simulink model "mpc555_v12_sade_ve_duzenli"  (Simulink 7.0)
settings: Solver=FixedStepDiscrete  StartTime=0.0  StopTime=inf  FixedStep=dt_sys  RelTol=1e-3
PreLoadFcn:
  | RTWConfigurationCB('preloadfcn', bdroot);
InitFcn:
  | % START RTW CONFIGURATION CODE %
  | RTWConfigurationCB('rtw_target_initfcn',gcs);
  | % END RTW CONFIGURATION CODE %
values from neighbouring files (symbols this model uses):
  dt = 1/50    (= 0.02)    [init_par.m]
  dt_serial_RX1 = dt/120    (= 0.000166666666667)    [init_par.m]
  dt_serial_TX2 = dt/120    (= 0.000166666666667)    [init_par.m]
undefined symbols (not defined in the file or in its folder): DiscIntNeverNeededParam
libraries: aerolibconvert2 x9, mpc555drivers x5, simulink x1
(part 1 of 2)
settings Model: Creator=PC  LastModifiedBy=eg
settings OptimizationCC: OptimizeModelRefInitCode=on  LifeSpan=1
settings DebuggingCC: AlgebraicLoopMsg=none
settings HardwareCC: ProdIntDivRoundTo=Zero  ProdEndianess=BigEndian  ProdHWDeviceType=Motorola PowerPC
settings RTWCC: SystemTargetFile=mpc555rt.tlc  TemplateMakefile=mpc555rt.tmf  Description=Target for Freescale MPC5xx (real-time)  ProcessScript=mpc555rt_make_rtw_hook
settings CodeAppCC: IgnoreCustomStorageClasses=off
settings STFCustomTargetCC: TargetLibSuffix=.a  TargetPreCompLibLocation=C:\MATLAB\R2007b\toolbox\rtw\targets\mpc555dk\drivers\lib\CODE_WARRIOR  GenFloatMathFcnCalls=ANSI_C  IncludeMdlTerminateFcn=off  CombineOutputUpdateFcns=on  ERTCustomFileBanners=on  SupportNonFinite=off  SupportContinuousTime=off  SupportNonInlinedSFcns=off  SystemTargetFile=mpc555rt.tlc
settings ERTTargetCC: TargetPreCompLibLocation=C:\MATLAB\R2007b\toolbox\rtw\targets\mpc555dk\drivers\lib\CODE_WARRIOR  GenFloatMathFcnCalls=ANSI_C  CompOptLevelCompliant=off  IncludeMdlTerminateFcn=off  SupportNonFinite=off  ModelStepFunctionPrototypeControlCompliant=off  ExtModeMexFile=MPC5xxExternalModeOpen  ExtModeIntrfLevel=Level2 - Open  InlinedParameterPlacement=NonHierarchical  ERTCustomFileTemplate=example_file_process.tlc
settings CustomProperty: DataType=RTWOptions_EnumType__toolbox_rtw_targets_mpc555dk_mpc555dk_mpc555rt_MPC555_OPTIMIZATION_SWITCH  Value=speed
settings EnumStrPairs: String=speed

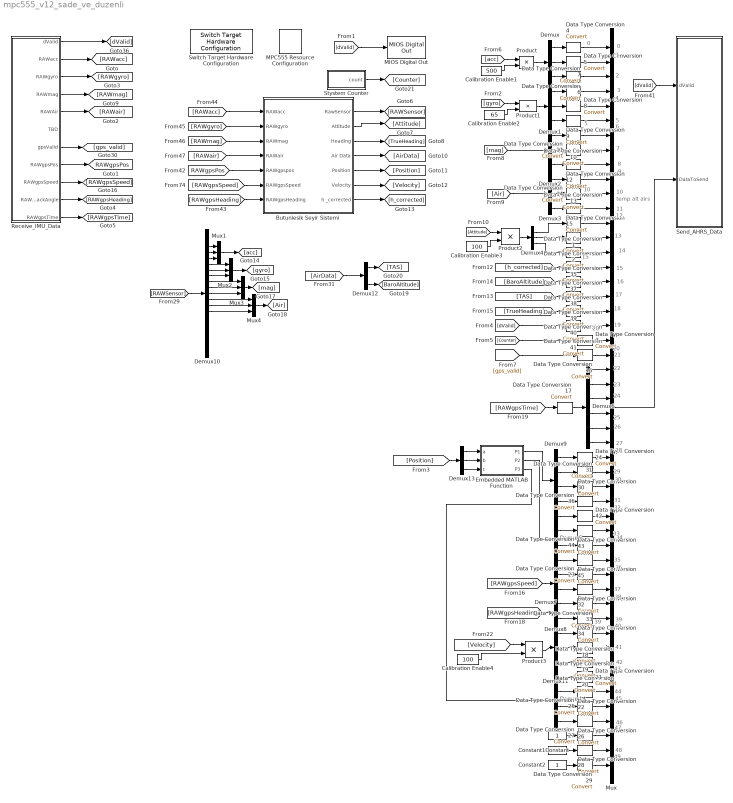
== system mpc555_v12_sade_ve_duzenli ==
  note: 0
  note: 5
  note: 10
  note: 15
  note: 20
  note: 39
  note: 27
  note: 0
  note: 1
  note: 2
  note: 4
  note: 5
  note: 6
  note: 7
  note: 8
  note: 9
  note: 10
  note: 11
  note: 12
  note: 13
  note: 14
  note: 15
  note: 16
  note: 3
  note: 17
  note: 18
  note: 19
  note: 20
  note: 21
  note: 22
  note: 23
  note: 24
  note: 25
  note: 26
  note: 28
  note: 29
  note: 30
  note: 31
  note: 32
  note: 33
  note: 34
  note: 35
  note: 36
  note: 37
  note: 38
  note: 39
  note: 40
  note: 41
  note: 42
  note: 43
  note: 44
  note: 45
  note: 46
  note: 47
  note: 48
  note: 49
  note: temp
      | alt
      | airs
  Butunlesik Seyir Sistemi : Subsystem
  Calibration Enable1 : Constant  Value=500  OutDataType=fixdt(1, 16)  OutScaling=2^0
  Calibration Enable2 : Constant  Value=65  OutDataType=fixdt(1, 16)  OutScaling=2^0
  Calibration Enable3 : Constant  Value=100  OutDataType=fixdt(1, 16)  OutScaling=2^0
  Calibration Enable4 : Constant  Value=100  OutDataType=fixdt(1, 16)  OutScaling=2^0
  Constant : Constant  OutDataType=sfix(16)  OutScaling=2^0
  Constant1 : Constant  OutDataType=sfix(16)  OutScaling=2^0
  Constant2 : Constant  OutDataType=sfix(16)  OutScaling=2^0
  Data Type Conversion{1..45} (45 alike) : DataTypeConversion  OutDataTypeMode=int16  OutDataType=sfix(16)  OutScaling=2^0
  Demux{,1..4,11,13} (7 alike) : Demux  Outputs=3
  Demux10 : Demux  Outputs=17
  Demux{5,9,12,14} (4 alike) : Demux
  Demux6 : Demux  Outputs=6
  Demux7 : Demux  Outputs=2
  Demux8 : Demux  Outputs=2
  Embedded MATLAB Function : Stateflow chart
  MIOS Digital Out : mpc555drivers/Modular Input//Output System (MIOS1)/MIOS Digital Out  SystemSampleTime=-1  bits=[3]  init=0  t=-1  enablePassThru=off
  MPC555 Resource Configuration : mpc555drivers/MPC555 Resource Configuration  Tag=RTW CONFIGURATION BLOCK  Priority=-100000  SystemSampleTime=-1  oldParentName=mpc555_v12_sade_ve_duzenli  oldBlockName=|
      | mpc555_v12_sade_ve_duzenli/MPC555
      | Resource
      | Configuration
  Mux : Mux  Inputs=50
  Mux{1..4} (4 alike) : Mux  Inputs=3
  Product{,1..3} (4 alike) : Product  OutDataType=sfix(16)  OutScaling=2^0  RndMeth=Zero
      mask Display: text(0.5, 0.5, ['SCI' num2str(module) '\nTransmit'],'horizontalAlignment','center'); port_label('input',1,'Data'); port_label('input', 2, 'Req');
  Receive_IMU_Data : Subsystem
  Send_AHRS_Data : Subsystem
  Stystem Counter : Stateflow chart
  Switch Target Hardware Configuration : mpc555drivers/Utilities/Switch Target Hardware Configuration  SystemSampleTime=-1
  tag scope: RAWgpsPos=global
  wires:
  Mux/1 -> Send_AHRS_Data/2(DataToSend)
  Data Type Conversion4/1 -> Mux/1
  Data Type Conversion5/1 -> Mux/2
  Data Type Conversion6/1 -> Mux/3
  Data Type Conversion7/1 -> Mux/4
  Data Type Conversion8/1 -> Mux/5
  Data Type Conversion9/1 -> Mux/6
  Data Type Conversion10/1 -> Mux/7
  Data Type Conversion11/1 -> Mux/8
  Data Type Conversion12/1 -> Mux/9
  Data Type Conversion13/1 -> Mux/10
  Data Type Conversion14/1 -> Mux/11
  Data Type Conversion15/1 -> Mux/12
  Data Type Conversion3/1 -> Mux/21
  Data Type Conversion16/1 -> Mux/22
  Demux6/2 -> Mux/24
  Data Type Conversion37/1 -> Mux/16
  Data Type Conversion38/1 -> Mux/17
  Data Type Conversion39/1 -> Mux/18
  Data Type Conversion40/1 -> Mux/19
  Data Type Conversion41/1 -> Mux/20
  Data Type Conversion23/1 -> Mux/37
  Data Type Conversion32/1 -> Mux/38
  Data Type Conversion33/1 -> Mux/39
  Data Type Conversion34/1 -> Mux/40
  [dValid] -> Send_AHRS_Data/1(dValid)
  Receive_IMU_Data/1(dValid) -> [dValid]
  Receive_IMU_Data/7(gpsValid) -> [gps_valid]
  Receive_IMU_Data/2(RAWacc) -> [RAWacc]
  Receive_IMU_Data/3(RAWgyro) -> [RAWgyro]
  Receive_IMU_Data/4(RAWmag) -> [RAWmag]
  Receive_IMU_Data/5(RAWAir) -> [RAWair]
  Receive_IMU_Data/8(RAWgpsPos) -> [RAWgpsPos]
  Receive_IMU_Data/9(RAWgpsSpeed) -> [RAWgpsSpeed]
  Receive_IMU_Data/10(RAWgpsTrackAngle) -> [RAWgpsHeading]
  Receive_IMU_Data/11(RAWgpsTime) -> [RAWgpsTime]
  Demux/1 -> Data Type Conversion4/1
  Demux/2 -> Data Type Conversion5/1
  [Air] -> Demux3/1
  Demux1/1 -> Data Type Conversion7/1
  Demux1/2 -> Data Type Conversion8/1
  Demux1/3 -> Data Type Conversion9/1
  Demux3/1 -> Data Type Conversion13/1
  Demux3/2 -> Data Type Conversion14/1
  Demux3/3 -> Data Type Conversion15/1
  Data Type Conversion1/1 -> Mux/13
  Data Type Conversion2/1 -> Mux/14
  Data Type Conversion35/1 -> Mux/15
  Demux4/1 -> Data Type Conversion1/1
  Demux4/2 -> Data Type Conversion2/1
  Demux4/3 -> Data Type Conversion35/1
  [RAWgpsHeading] -> Demux8/1
  Demux8/2 -> Data Type Conversion34/1
  Demux8/1 -> Data Type Conversion33/1
  Demux7/2 -> Data Type Conversion32/1
  Demux7/1 -> Data Type Conversion23/1
  [RAWgpsSpeed] -> Demux7/1
  Demux6/6 -> Mux/28
  Demux6/5 -> Mux/27
  Demux6/4 -> Mux/26
  Demux6/3 -> Mux/25
  [RAWgpsTime] -> Data Type Conversion17/1
  [h_corrected] -> Data Type Conversion37/1
  [BaroAltitude] -> Data Type Conversion38/1
  [TAS] -> Data Type Conversion39/1
  [dValid] -> Data Type Conversion41/1
  Product2/1 -> Demux4/1
  [Attitude] -> Product2/1
  Calibration Enable3/1 -> Product2/2
  Demux9/1 -> Data Type Conversion24/1
  Demux9/2 -> Data Type Conversion30/1
  Demux9/3 -> Data Type Conversion31/1
  Demux9/4 -> Data Type Conversion36/1
  Demux5/2 -> Data Type Conversion43/1
  Demux5/3 -> Data Type Conversion44/1
  Demux5/4 -> Data Type Conversion45/1
  Data Type Conversion17/1 -> Demux6/1
  Demux6/1 -> Mux/23
  Data Type Conversion18/1 -> Mux/41
  Data Type Conversion19/1 -> Mux/42
  Data Type Conversion20/1 -> Mux/43
  Data Type Conversion21/1 -> Mux/44
  Data Type Conversion22/1 -> Mux/45
  Data Type Conversion25/1 -> Mux/46
  Data Type Conversion26/1 -> Mux/47
  [RAWacc] -> Butunlesik Seyir Sistemi/1(RAWacc)
  [RAWgyro] -> Butunlesik Seyir Sistemi/2(RAWgyro)
  [RAWmag] -> Butunlesik Seyir Sistemi/3(RAWmag)
  [RAWair] -> Butunlesik Seyir Sistemi/4(RAWair)
  [RAWgpsPos] -> Butunlesik Seyir Sistemi/5(RAWgpspos)
  [RAWgpsSpeed] -> Butunlesik Seyir Sistemi/6(RAWgpsSpeed)
  [RAWgpsHeading] -> Butunlesik Seyir Sistemi/7(RAWgpsHeading)
  Butunlesik Seyir Sistemi/1(RawSensor) -> [RAWSensor]
  Butunlesik Seyir Sistemi/2(Attitude) -> [Attitude]
  Butunlesik Seyir Sistemi/3(Heading) -> [TrueHeading]
  Butunlesik Seyir Sistemi/4(Air Data) -> [AirData]
  Butunlesik Seyir Sistemi/5(Position) -> [Position]
  Butunlesik Seyir Sistemi/6(Velocity) -> [Velocity]
  Butunlesik Seyir Sistemi/7(h _corrected) -> [h_corrected]
  [RAWSensor] -> Demux10/1
  Demux10/1 -> Mux1/1
  Demux10/2 -> Mux1/2
  Demux10/3 -> Mux1/3
  Mux1/1 -> [acc]
  Mux2/1 -> [gyro]
  Demux10/4 -> Mux2/1
  Demux10/5 -> Mux2/2
  Demux10/6 -> Mux2/3
  Mux3/1 -> [mag]
  Demux10/7 -> Mux3/1
  Demux10/8 -> Mux3/2
  Demux10/9 -> Mux3/3
  Mux4/1 -> [Air]
  Demux10/10 -> Mux4/1
  Demux10/11 -> Mux4/2
  Demux10/12 -> Mux4/3
  [AirData] -> Demux12/1
  Demux12/4 -> [BaroAltitude]
  Demux12/1 -> [TAS]
  Data Type Conversion27/1 -> Mux/48
  Data Type Conversion28/1 -> Mux/49
  Data Type Conversion29/1 -> Mux/50
  [dValid] -> MIOS Digital Out/1
  Demux/3 -> Data Type Conversion6/1
  Product/1 -> Demux/1
  [acc] -> Product/1
  Calibration Enable1/1 -> Product/2
  [gyro] -> Product1/1
  Calibration Enable2/1 -> Product1/2
  Product1/1 -> Demux1/1
  Demux2/1 -> Data Type Conversion10/1
  Demux2/2 -> Data Type Conversion11/1
  Demux2/3 -> Data Type Conversion12/1
  Embedded MATLAB Function/1(P1) -> Demux9/1
  Embedded MATLAB Function/2(P2) -> Demux5/1
  Demux5/1 -> Data Type Conversion42/1
  [Velocity] -> Product3/1
  Calibration Enable4/1 -> Product3/2
  Product3/1 -> Demux11/1
  Data Type Conversion24/1 -> Mux/29
  Data Type Conversion30/1 -> Mux/30
  Data Type Conversion31/1 -> Mux/31
  Data Type Conversion36/1 -> Mux/32
  Data Type Conversion42/1 -> Mux/33
  Data Type Conversion43/1 -> Mux/34
  Data Type Conversion44/1 -> Mux/35
  Data Type Conversion45/1 -> Mux/36
  [Position] -> Demux13/1
  Demux11/1 -> Data Type Conversion18/1
  Demux11/2 -> Data Type Conversion19/1
  Demux11/3 -> Data Type Conversion20/1
  Stystem Counter/1(count) -> [Counter]
  [Counter] -> Data Type Conversion3/1
  [gps_valid] -> Data Type Conversion16/1
  Embedded MATLAB Function/3(P3) -> Demux14/1
  Demux14/1 -> Data Type Conversion21/1
  Demux14/2 -> Data Type Conversion22/1
  Demux14/3 -> Data Type Conversion25/1
  Demux14/4 -> Data Type Conversion26/1
  Constant/1 -> Data Type Conversion27/1
  Constant1/1 -> Data Type Conversion28/1
  Constant2/1 -> Data Type Conversion29/1
  Demux13/2 -> Embedded MATLAB Function/2(b)
  [mag] -> Demux2/1
  Demux13/1 -> Embedded MATLAB Function/1(a)
  Demux13/3 -> Embedded MATLAB Function/3(c)
  [TrueHeading] -> Data Type Conversion40/1

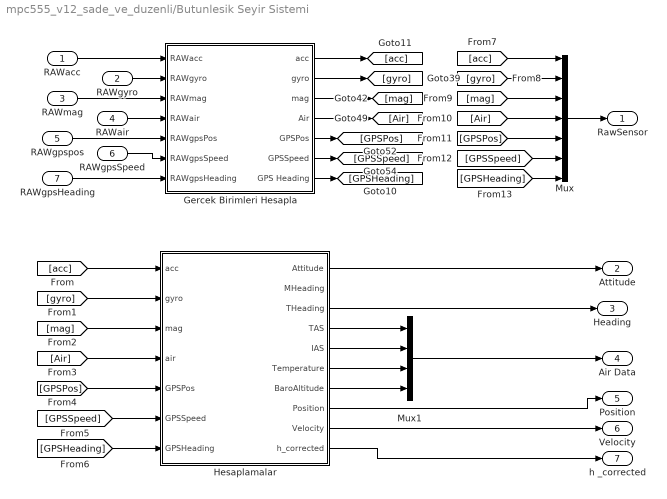
== system mpc555_v12_sade_ve_duzenli/Butunlesik Seyir Sistemi ==
  RAWacc : Inport  OutDataType=fixdt(1, 16)  OutScaling=2^0
  RAWgyro : Inport  Port=2  OutDataType=fixdt(1, 16)  OutScaling=2^0
  RAWmag : Inport  Port=3  OutDataType=fixdt(1, 16)  OutScaling=2^0
  RAWair : Inport  Port=4  OutDataType=fixdt(1, 16)  OutScaling=2^0
  RAWgpspos : Inport  Port=5  OutDataType=fixdt(1, 16)  OutScaling=2^0
  RAWgpsSpeed : Inport  Port=6  OutDataType=fixdt(1, 16)  OutScaling=2^0
  RAWgpsHeading : Inport  Port=7  OutDataType=fixdt(1, 16)  OutScaling=2^0
  Gercek Birimleri Hesapla : Subsystem
  Hesaplamalar : Subsystem
  Mux : Mux  Inputs=7
  Mux1 : Mux
  RawSensor : Outport
  Attitude : Outport  Port=2  OutDataType=fixdt(1, 16)  OutScaling=2^0
  Heading : Outport  Port=3  OutDataType=fixdt(1, 16)  OutScaling=2^0
  Air Data : Outport  Port=4  OutDataType=fixdt(1, 16)  OutScaling=2^0
  Position : Outport  Port=5  OutDataType=fixdt(1, 16)  OutScaling=2^0
  Velocity : Outport  Port=6  OutDataType=fixdt(1, 16)  OutScaling=2^0
  h _corrected : Outport  Port=7  OutDataType=fixdt(1, 16)  OutScaling=2^0
  wires:
  Gercek Birimleri Hesapla/1(acc) -> [acc]
  Gercek Birimleri Hesapla/2(gyro) -> [gyro]
  Gercek Birimleri Hesapla/3(mag) -> [mag]
  Gercek Birimleri Hesapla/4(Air) -> [Air]
  Gercek Birimleri Hesapla/5(GPSPos) -> [GPSPos]
  Gercek Birimleri Hesapla/6(GPSSpeed) -> [GPSSpeed]
  Gercek Birimleri Hesapla/7(GPS Heading) -> [GPSHeading]
  RAWacc/1 -> Gercek Birimleri Hesapla/1(RAWacc)
  RAWgyro/1 -> Gercek Birimleri Hesapla/2(RAWgyro)
  RAWmag/1 -> Gercek Birimleri Hesapla/3(RAWmag)
  RAWair/1 -> Gercek Birimleri Hesapla/4(RAWair)
  RAWgpspos/1 -> Gercek Birimleri Hesapla/5(RAWgpsPos)
  RAWgpsSpeed/1 -> Gercek Birimleri Hesapla/6(RAWgpsSpeed)
  RAWgpsHeading/1 -> Gercek Birimleri Hesapla/7(RAWgpsHeading)
  [acc] -> Mux/1
  [gyro] -> Mux/2
  [Air] -> Mux/4
  [GPSPos] -> Mux/5
  [GPSSpeed] -> Mux/6
  [GPSHeading] -> Mux/7
  [acc] -> Hesaplamalar/1(acc)
  [gyro] -> Hesaplamalar/2(gyro)
  [mag] -> Hesaplamalar/3(mag)
  [Air] -> Hesaplamalar/4(air)
  [GPSPos] -> Hesaplamalar/5(GPSPos)
  [GPSSpeed] -> Hesaplamalar/6(GPSSpeed)
  [GPSHeading] -> Hesaplamalar/7(GPSHeading)
  Mux/1 -> RawSensor/1
  Hesaplamalar/4(TAS) -> Mux1/1
  Hesaplamalar/5(IAS) -> Mux1/2
  Hesaplamalar/6(Temperature) -> Mux1/3
  Hesaplamalar/7(BaroAltitude) -> Mux1/4
  Mux1/1 -> Air Data/1
  Hesaplamalar/3(THeading) -> Heading/1
  Hesaplamalar/8(Position) -> Position/1
  Hesaplamalar/9(Velocity) -> Velocity/1
  Hesaplamalar/10(h_corrected) -> h _corrected/1
  Hesaplamalar/1(Attitude) -> Attitude/1
  [mag] -> Mux/3

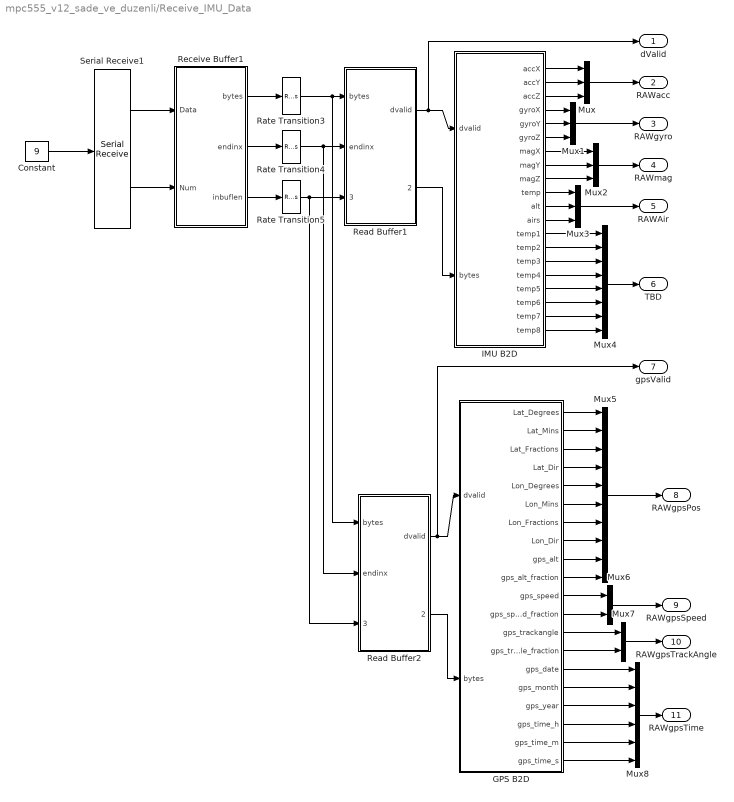
== system mpc555_v12_sade_ve_duzenli/Receive_IMU_Data ==
  Constant : Constant  Value=9  OutDataTypeMode=uint32  OutDataType=sfix(16)  OutScaling=2^0  SampleTime=dt_serial_RX1
  GPS B2D : Stateflow chart  TreatAsAtomicUnit=on
  IMU B2D : Stateflow chart  TreatAsAtomicUnit=on
  Mux{,1..3} (4 alike) : Mux  Inputs=3
  Mux4 : Mux  Inputs=8
  Mux5 : Mux  Inputs=10
  Mux6 : Mux  Inputs=2
  Mux7 : Mux  Inputs=2
  Mux8 : Mux  Inputs=6
  Rate Transition3 : RateTransition  OutPortSampleTime=dt
  Rate Transition4 : RateTransition  OutPortSampleTime=dt
  Rate Transition5 : RateTransition  OutPortSampleTime=dt
  Read Buffer1 : Stateflow chart  TreatAsAtomicUnit=on
  Read Buffer2 : Stateflow chart  TreatAsAtomicUnit=on
  Receive Buffer1 : Stateflow chart  TreatAsAtomicUnit=on
  Serial Receive1 : mpc555drivers/Serial Communications Interface (SCI)/Serial Receive  module=1  show_length=on  max_length=9  show_reset=off  show_bytes_read=on  show_flags=off  show_overrun=off  T=dt_serial_RX1
  dValid : Outport  OutDataType=sfix(16)  OutScaling=2^0
  RAWacc : Outport  Port=2  OutDataType=sfix(16)  OutScaling=2^0
  RAWgyro : Outport  Port=3  OutDataType=sfix(16)  OutScaling=2^0
  RAWmag : Outport  Port=4  OutDataType=sfix(16)  OutScaling=2^0
  RAWAir : Outport  Port=5  OutDataType=sfix(16)  OutScaling=2^0
  TBD : Outport  Port=6  OutDataType=sfix(16)  OutScaling=2^0
  gpsValid : Outport  Port=7  OutDataType=sfix(16)  OutScaling=2^0
  RAWgpsPos : Outport  Port=8  OutDataType=sfix(16)  OutScaling=2^0
  RAWgpsSpeed : Outport  Port=9  OutDataType=sfix(16)  OutScaling=2^0
  RAWgpsTrackAngle : Outport  Port=10  OutDataType=sfix(16)  OutScaling=2^0
  RAWgpsTime : Outport  Port=11  OutDataType=sfix(16)  OutScaling=2^0
  wires:
  Rate Transition3/1 -> Read Buffer1/1(bytes), Read Buffer2/1(bytes)
  Receive Buffer1/1(bytes) -> Rate Transition3/1
  Receive Buffer1/2(endinx) -> Rate Transition4/1
  Receive Buffer1/3(inbuflen) -> Rate Transition5/1
  Rate Transition4/1 -> Read Buffer1/2(endinx), Read Buffer2/2(endinx)
  Rate Transition5/1 -> Read Buffer1/3(inbuflenSC2), Read Buffer2/3(inbuflenSC2)
  Serial Receive1/1 -> Receive Buffer1/1(Data)
  Serial Receive1/2 -> Receive Buffer1/2(Num)
  Constant/1 -> Serial Receive1/1
  Read Buffer1/1(dvalid) -> IMU B2D/1(dvalid), dValid/1
  Read Buffer1/2(imu_data) -> IMU B2D/2(bytes)
  Read Buffer2/1(dvalid) -> gpsValid/1, GPS B2D/1(dvalid)
  Read Buffer2/2(imu_data) -> GPS B2D/2(bytes)
  IMU B2D/1(accX) -> Mux/1
  IMU B2D/2(accY) -> Mux/2
  IMU B2D/3(accZ) -> Mux/3
  Mux/1 -> RAWacc/1
  IMU B2D/4(gyroX) -> Mux1/1
  IMU B2D/5(gyroY) -> Mux1/2
  IMU B2D/6(gyroZ) -> Mux1/3
  Mux1/1 -> RAWgyro/1
  IMU B2D/7(magX) -> Mux2/1
  IMU B2D/8(magY) -> Mux2/2
  IMU B2D/9(magZ) -> Mux2/3
  Mux2/1 -> RAWmag/1
  IMU B2D/10(temp) -> Mux3/1
  IMU B2D/11(alt) -> Mux3/2
  IMU B2D/12(airs) -> Mux3/3
  Mux3/1 -> RAWAir/1
  IMU B2D/13(temp1) -> Mux4/1
  IMU B2D/14(temp2) -> Mux4/2
  IMU B2D/15(temp3) -> Mux4/3
  IMU B2D/16(temp4) -> Mux4/4
  IMU B2D/17(temp5) -> Mux4/5
  IMU B2D/18(temp6) -> Mux4/6
  IMU B2D/19(temp7) -> Mux4/7
  IMU B2D/20(temp8) -> Mux4/8
  Mux4/1 -> TBD/1
  GPS B2D/1(Lat_Degrees) -> Mux5/1
  GPS B2D/2(Lat_Mins) -> Mux5/2
  GPS B2D/3(Lat_Fractions) -> Mux5/3
  GPS B2D/4(Lat_Dir) -> Mux5/4
  GPS B2D/5(Lon_Degrees) -> Mux5/5
  GPS B2D/6(Lon_Mins) -> Mux5/6
  GPS B2D/7(Lon_Fractions) -> Mux5/7
  GPS B2D/8(Lon_Dir) -> Mux5/8
  GPS B2D/9(gps_alt) -> Mux5/9
  GPS B2D/10(gps_alt_fraction) -> Mux5/10
  Mux5/1 -> RAWgpsPos/1
  GPS B2D/11(gps_speed) -> Mux6/1
  GPS B2D/12(gps_speed_fraction) -> Mux6/2
  Mux6/1 -> RAWgpsSpeed/1
  GPS B2D/13(gps_trackangle) -> Mux7/1
  GPS B2D/14(gps_trackangle_fraction) -> Mux7/2
  Mux7/1 -> RAWgpsTrackAngle/1
  GPS B2D/15(gps_date) -> Mux8/1
  GPS B2D/16(gps_month) -> Mux8/2
  GPS B2D/17(gps_year) -> Mux8/3
  GPS B2D/18(gps_time_h) -> Mux8/4
  GPS B2D/19(gps_time_m) -> Mux8/5
  GPS B2D/20(gps_time_s) -> Mux8/6
  Mux8/1 -> RAWgpsTime/1

== system mpc555_v12_sade_ve_duzenli/Send_AHRS_Data ==
  dValid : Inport  OutDataType=sfix(16)  OutScaling=2^0
  DataToSend : Inport  Port=2  OutDataType=sfix(16)  OutScaling=2^0
  Put in array : Stateflow chart  TreatAsAtomicUnit=on
  Rate Transition13 : RateTransition  OutPortSampleTime=dt_serial_TX2
  Rate Transition14 : RateTransition  OutPortSampleTime=dt_serial_TX2
  Transmit2 : Subsystem
  wires:
  Put in array/1(bytes1) -> Rate Transition13/1
  Rate Transition13/1 -> Transmit2/1(outbytes)
  Rate Transition14/1 -> Transmit2/2(outsync)
  Put in array/2(sync) -> Rate Transition14/1
  dValid/1 -> Put in array/1(dvalid)
  DataToSend/1 -> Put in array/2(bytes)

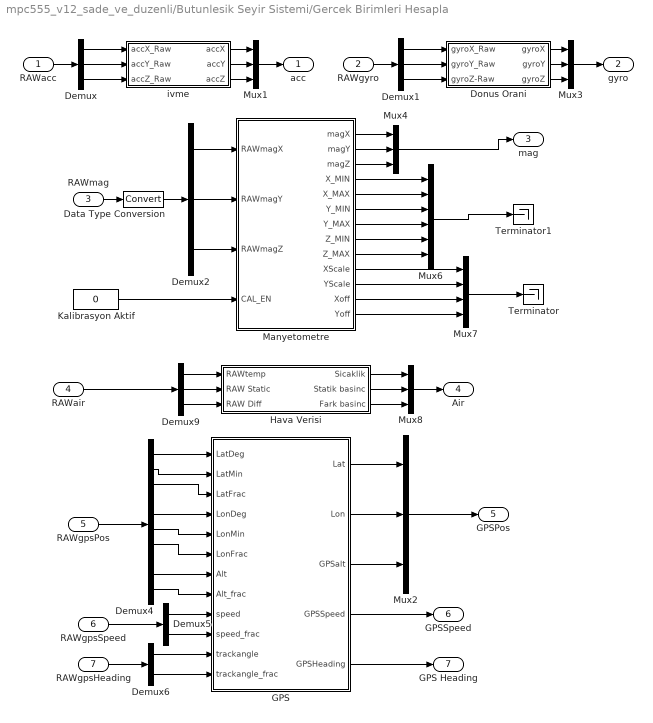
== system mpc555_v12_sade_ve_duzenli/Butunlesik Seyir Sistemi/Gercek Birimleri Hesapla ==
  RAWacc : Inport  OutDataType=sfix(16)  OutScaling=2^0
  RAWgyro : Inport  Port=2  OutDataType=sfix(16)  OutScaling=2^0
  RAWmag : Inport  Port=3  OutDataType=sfix(16)  OutScaling=2^0
  RAWair : Inport  Port=4  OutDataType=sfix(16)  OutScaling=2^0
  RAWgpsPos : Inport  Port=5  OutDataType=sfix(16)  OutScaling=2^0
  RAWgpsSpeed : Inport  Port=6  OutDataType=sfix(16)  OutScaling=2^0
  RAWgpsHeading : Inport  Port=7  OutDataType=sfix(16)  OutScaling=2^0
  Data Type Conversion : DataTypeConversion  OutDataTypeMode=double  OutDataType=fixdt(1, 16)  OutScaling=2^0
  Demux{,1..2,9} (4 alike) : Demux  Outputs=3
  Demux4 : Demux  Outputs=10
  Demux5 : Demux  Outputs=2
  Demux6 : Demux  Outputs=2
  Donus Orani : Subsystem
  GPS : Stateflow chart  TreatAsAtomicUnit=on
  Hava Verisi : Subsystem
  Kalibrasyon Aktif : Constant  Value=0  OutDataType=fixdt(1, 16)  OutScaling=2^0
  Manyetometre : Stateflow chart  TreatAsAtomicUnit=on
  Mux{1..4,8} (5 alike) : Mux  Inputs=3
  Mux6 : Mux  Inputs=6
  Mux7 : Mux
  Terminator : Terminator
  Terminator1 : Terminator
  ivme : Subsystem
  acc : Outport  OutDataType=fixdt(1, 16)  OutScaling=2^0
  gyro : Outport  Port=2  OutDataType=fixdt(1, 16)  OutScaling=2^0
  mag : Outport  Port=3  OutDataType=fixdt(1, 16)  OutScaling=2^0
  Air : Outport  Port=4  OutDataType=fixdt(1, 16)  OutScaling=2^0
  GPSPos : Outport  Port=5  OutDataType=fixdt(1, 16)  OutScaling=2^0
  GPSSpeed : Outport  Port=6  OutDataType=fixdt(1, 16)  OutScaling=2^0
  GPS Heading : Outport  Port=7  OutDataType=fixdt(1, 16)  OutScaling=2^0
  wires:
  GPS/5(GPSHeading) -> GPS Heading/1
  GPS/4(GPSSpeed) -> GPSSpeed/1
  Mux2/1 -> GPSPos/1
  GPS/3(GPSalt) -> Mux2/3
  GPS/2(Lon) -> Mux2/2
  GPS/1(Lat) -> Mux2/1
  RAWgpsSpeed/1 -> Demux5/1
  RAWgpsHeading/1 -> Demux6/1
  Demux6/2 -> GPS/12(trackangle_frac)
  Demux6/1 -> GPS/11(trackangle)
  Demux5/2 -> GPS/10(speed_frac)
  Demux5/1 -> GPS/9(speed)
  Demux4/10 -> GPS/8(Alt_frac)
  Demux4/9 -> GPS/7(Alt)
  Demux4/7 -> GPS/6(LonFrac)
  Demux4/6 -> GPS/5(LonMin)
  Demux4/5 -> GPS/4(LonDeg)
  Demux4/3 -> GPS/3(LatFrac)
  Demux4/2 -> GPS/2(LatMin)
  Demux4/1 -> GPS/1(LatDeg)
  RAWgpsPos/1 -> Demux4/1
  RAWmag/1 -> Data Type Conversion/1
  Mux4/1 -> mag/1
  Manyetometre/3(magZ) -> Mux4/3
  Manyetometre/2(magY) -> Mux4/2
  Manyetometre/1(magX) -> Mux4/1
  Demux2/3 -> Manyetometre/3(RAWmagZ)
  Demux2/2 -> Manyetometre/2(RAWmagY)
  Demux2/1 -> Manyetometre/1(RAWmagX)
  Mux3/1 -> gyro/1
  Donus Orani/3(gyroZ) -> Mux3/3
  Donus Orani/2(gyroY) -> Mux3/2
  Donus Orani/1(gyroX) -> Mux3/1
  RAWgyro/1 -> Demux1/1
  Demux1/3 -> Donus Orani/3(gyroZ-Raw)
  Demux1/2 -> Donus Orani/2(gyroY_Raw)
  Demux1/1 -> Donus Orani/1(gyroX_Raw)
  Mux1/1 -> acc/1
  ivme/3(accZ) -> Mux1/3
  ivme/2(accY) -> Mux1/2
  ivme/1(accX) -> Mux1/1
  RAWacc/1 -> Demux/1
  Demux/3 -> ivme/3(accZ_Raw)
  Demux/2 -> ivme/2(accY_Raw)
  Demux/1 -> ivme/1(accX_Raw)
  Data Type Conversion/1 -> Demux2/1
  Kalibrasyon Aktif/1 -> Manyetometre/4(CAL_EN)
  Manyetometre/4(X_MIN) -> Mux6/1
  Manyetometre/5(X_MAX) -> Mux6/2
  Manyetometre/6(Y_MIN) -> Mux6/3
  Manyetometre/7(Y_MAX) -> Mux6/4
  Manyetometre/8(Z_MIN) -> Mux6/5
  Manyetometre/9(Z_MAX) -> Mux6/6
  Manyetometre/10(XScale) -> Mux7/1
  Manyetometre/11(YScale) -> Mux7/2
  Manyetometre/12(Xoff) -> Mux7/3
  Manyetometre/13(Yoff) -> Mux7/4
  Hava Verisi/1(Sicaklik) -> Mux8/1
  Hava Verisi/2(Statik basinc) -> Mux8/2
  Hava Verisi/3(Fark basinc) -> Mux8/3
  Demux9/1 -> Hava Verisi/1(RAWtemp)
  Demux9/2 -> Hava Verisi/2(RAW Static)
  Demux9/3 -> Hava Verisi/3(RAW Diff)
  RAWair/1 -> Demux9/1
  Mux8/1 -> Air/1
  Mux7/1 -> Terminator/1
  Mux6/1 -> Terminator1/1

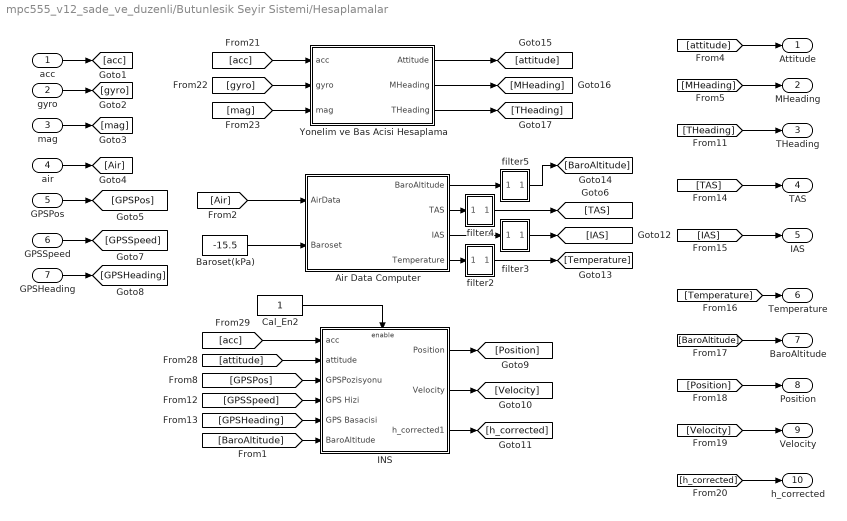
== system mpc555_v12_sade_ve_duzenli/Butunlesik Seyir Sistemi/Hesaplamalar ==
  acc : Inport  OutDataType=fixdt(1, 16)  OutScaling=2^0
  gyro : Inport  Port=2  OutDataType=fixdt(1, 16)  OutScaling=2^0
  mag : Inport  Port=3  OutDataType=fixdt(1, 16)  OutScaling=2^0
  air : Inport  Port=4  OutDataType=fixdt(1, 16)  OutScaling=2^0
  GPSPos : Inport  Port=5  OutDataType=fixdt(1, 16)  OutScaling=2^0
  GPSSpeed : Inport  Port=6  OutDataType=fixdt(1, 16)  OutScaling=2^0
  GPSHeading : Inport  Port=7  OutDataType=fixdt(1, 16)  OutScaling=2^0
  Air Data Computer : Stateflow chart  TreatAsAtomicUnit=on
  Baroset(kPa) : Constant  Value=-15.5  OutDataType=fixdt(1, 16)  OutScaling=2^0
  Cal_En2 : Constant  OutDataType=fixdt(1, 16)  OutScaling=2^0
  INS : Subsystem
  Yonelim ve Bas Acisi Hesaplama : Subsystem
  filter2 : Stateflow chart  TreatAsAtomicUnit=on
  filter3 : Stateflow chart  TreatAsAtomicUnit=on
  filter4 : Stateflow chart  TreatAsAtomicUnit=on
  filter5 : Stateflow chart  TreatAsAtomicUnit=on
  Attitude : Outport  OutDataType=fixdt(1, 16)  OutScaling=2^0
  MHeading : Outport  Port=2  OutDataType=fixdt(1, 16)  OutScaling=2^0
  THeading : Outport  Port=3  OutDataType=fixdt(1, 16)  OutScaling=2^0
  TAS : Outport  Port=4  OutDataType=fixdt(1, 16)  OutScaling=2^0
  IAS : Outport  Port=5  OutDataType=fixdt(1, 16)  OutScaling=2^0
  Temperature : Outport  Port=6  OutDataType=fixdt(1, 16)  OutScaling=2^0
  BaroAltitude : Outport  Port=7  OutDataType=fixdt(1, 16)  OutScaling=2^0
  Position : Outport  Port=8  OutDataType=fixdt(1, 16)  OutScaling=2^0
  Velocity : Outport  Port=9  OutDataType=fixdt(1, 16)  OutScaling=2^0
  h_corrected : Outport  Port=10  OutDataType=fixdt(1, 16)  OutScaling=2^0
  wires:
  [attitude] -> INS/2(attitude)
  [acc] -> INS/1(acc)
  [GPSPos] -> INS/3(GPSPozisyonu)
  [GPSSpeed] -> INS/4(GPS Hizi)
  [GPSHeading] -> INS/5(GPS Basacisi)
  Cal_En2/1 -> INS/Enable
  [BaroAltitude] -> INS/6(BaroAltitude)
  [Air] -> Air Data Computer/1(AirData)
  Baroset(kPa)/1 -> Air Data Computer/2(Baroset)
  Air Data Computer/1(BaroAltitude) -> filter5/1(u)
  Air Data Computer/2(TAS) -> filter4/1(u)
  Air Data Computer/3(IAS) -> filter3/1(u)
  Air Data Computer/4(Temperature) -> filter2/1(u)
  filter2/1(y) -> [Temperature]
  filter3/1(y) -> [IAS]
  filter5/1(y) -> [BaroAltitude]
  acc/1 -> [acc]
  gyro/1 -> [gyro]
  mag/1 -> [mag]
  air/1 -> [Air]
  GPSPos/1 -> [GPSPos]
  GPSSpeed/1 -> [GPSSpeed]
  GPSHeading/1 -> [GPSHeading]
  [attitude] -> Attitude/1
  [MHeading] -> MHeading/1
  [THeading] -> THeading/1
  [TAS] -> TAS/1
  [IAS] -> IAS/1
  [Temperature] -> Temperature/1
  [BaroAltitude] -> BaroAltitude/1
  [Position] -> Position/1
  [Velocity] -> Velocity/1
  [h_corrected] -> h_corrected/1
  [acc] -> Yonelim ve Bas Acisi Hesaplama/1(acc)
  [gyro] -> Yonelim ve Bas Acisi Hesaplama/2(gyro)
  [mag] -> Yonelim ve Bas Acisi Hesaplama/3(mag)
  Yonelim ve Bas Acisi Hesaplama/1(Attitude) -> [attitude]
  Yonelim ve Bas Acisi Hesaplama/2(MHeading) -> [MHeading]
  Yonelim ve Bas Acisi Hesaplama/3(THeading) -> [THeading]
  INS/1(Position) -> [Position]
  INS/2(Velocity) -> [Velocity]
  INS/3(h_corrected1) -> [h_corrected]
  filter4/1(y) -> [TAS]

== system mpc555_v12_sade_ve_duzenli/Send_AHRS_Data/Transmit2 ==
  outbytes : Inport
  outsync : Inport  Port=2
  Serial Transmit : mpc555drivers/Serial Communications Interface (SCI)/Serial Transmit  module=2  show_length=on  show_num_sent=off  T=dt_serial_TX2
  Serialize : Stateflow chart  TreatAsAtomicUnit=on
  wires:
  Serialize/2(Req) -> Serial Transmit/2
  outsync/1 -> Serialize/2(sync)
  outbytes/1 -> Serialize/1(bytes)
  Serialize/1(Data) -> Serial Transmit/1

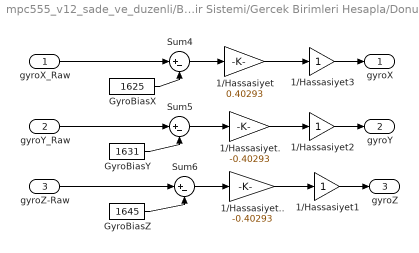
== system mpc555_v12_sade_ve_duzenli/Butunlesik Seyir Sistemi/Gercek Birimleri Hesapla/Donus Orani ==
  gyroX_Raw : Inport  OutDataType=sfix(16)  OutScaling=2^0
  gyroY_Raw : Inport  Port=2  OutDataType=sfix(16)  OutScaling=2^0
  gyroZ-Raw : Inport  Port=3  OutDataType=sfix(16)  OutScaling=2^0
  1/Hassasiyet : Gain  Gain=0.40293  ParameterDataType=fixdt(1, 16)  ParameterScaling=2^0  OutDataType=fixdt(1, 16)  OutScaling=2^0  SampleTime=dt
  1/Hassasiyet. : Gain  Gain=-0.40293  ParameterDataType=fixdt(1, 16)  ParameterScaling=2^0  OutDataType=fixdt(1, 16)  OutScaling=2^0  SampleTime=dt
  1/Hassasiyet.. : Gain  Gain=-0.40293  ParameterDataType=fixdt(1, 16)  ParameterScaling=2^0  OutDataType=fixdt(1, 16)  OutScaling=2^0  SampleTime=dt
  1/Hassasiyet1 : Gain  ParameterDataType=fixdt(1, 16)  ParameterScaling=2^0  OutDataType=fixdt(1, 16)  OutScaling=2^0  SampleTime=dt
  1/Hassasiyet2 : Gain  ParameterDataType=fixdt(1, 16)  ParameterScaling=2^0  OutDataType=fixdt(1, 16)  OutScaling=2^0  SampleTime=dt
  1/Hassasiyet3 : Gain  ParameterDataType=fixdt(1, 16)  ParameterScaling=2^0  OutDataType=fixdt(1, 16)  OutScaling=2^0  SampleTime=dt
  GyroBiasX : Constant  Value=1625  OutDataType=fixdt(1, 16)  OutScaling=2^0
  GyroBiasY : Constant  Value=1631  OutDataType=fixdt(1, 16)  OutScaling=2^0
  GyroBiasZ : Constant  Value=1645  OutDataType=fixdt(1, 16)  OutScaling=2^0
  Sum4 : Sum  Inputs=|+-  OutDataType=fixdt(1, 16)  OutScaling=2^0
  Sum5 : Sum  Inputs=|+-  OutDataType=fixdt(1, 16)  OutScaling=2^0
  Sum6 : Sum  Inputs=|+-  OutDataType=fixdt(1, 16)  OutScaling=2^0
  gyroX : Outport  OutDataType=fixdt(1, 16)  OutScaling=2^0
  gyroY : Outport  Port=2  OutDataType=fixdt(1, 16)  OutScaling=2^0
  gyroZ : Outport  Port=3  OutDataType=fixdt(1, 16)  OutScaling=2^0
  wires:
  gyroZ-Raw/1 -> Sum6/1
  gyroY_Raw/1 -> Sum5/1
  gyroX_Raw/1 -> Sum4/1
  1/Hassasiyet../1 -> 1/Hassasiyet1/1
  1/Hassasiyet./1 -> 1/Hassasiyet2/1
  Sum6/1 -> 1/Hassasiyet../1
  Sum5/1 -> 1/Hassasiyet./1
  1/Hassasiyet/1 -> 1/Hassasiyet3/1
  Sum4/1 -> 1/Hassasiyet/1
  GyroBiasZ/1 -> Sum6/2
  GyroBiasY/1 -> Sum5/2
  GyroBiasX/1 -> Sum4/2
  1/Hassasiyet1/1 -> gyroZ/1
  1/Hassasiyet2/1 -> gyroY/1
  1/Hassasiyet3/1 -> gyroX/1

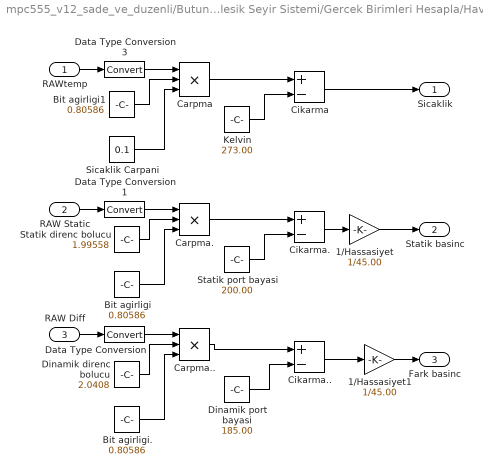
== system mpc555_v12_sade_ve_duzenli/Butunlesik Seyir Sistemi/Gercek Birimleri Hesapla/Hava Verisi ==
  RAWtemp : Inport  OutDataType=fixdt(1, 16)  OutScaling=2^0
  RAW Static : Inport  Port=2  OutDataType=fixdt(1, 16)  OutScaling=2^0
  RAW Diff : Inport  Port=3  OutDataType=fixdt(1, 16)  OutScaling=2^0
  1/Hassasiyet : Gain  Gain=1/45.00  ParameterDataType=fixdt(1, 16)  ParameterScaling=2^0  OutDataType=fixdt(1, 16)  OutScaling=2^0
  1/Hassasiyet1 : Gain  Gain=1/45.00  ParameterDataType=fixdt(1, 16)  ParameterScaling=2^0  OutDataType=fixdt(1, 16)  OutScaling=2^0
  Bit agirligi : Constant  Value=0.80586  OutDataType=fixdt(1, 16)  OutScaling=2^0
  Bit agirligi. : Constant  Value=0.80586  OutDataType=fixdt(1, 16)  OutScaling=2^0
  Bit agirligi1 : Constant  Value=0.80586  OutDataType=fixdt(1, 16)  OutScaling=2^0
  Carpma : Product  Inputs=3  OutDataType=fixdt(1, 16)  OutScaling=2^0  RndMeth=Zero
  Carpma. : Product  Inputs=3  OutDataType=fixdt(1, 16)  OutScaling=2^0  RndMeth=Zero
  Carpma.. : Product  Inputs=3  OutDataType=fixdt(1, 16)  OutScaling=2^0  RndMeth=Zero
  Cikarma : Sum  Inputs=+-  OutDataType=fixdt(1, 16)  OutScaling=2^-10
  Cikarma. : Sum  Inputs=+-  OutDataType=fixdt(1, 16)  OutScaling=2^-10
  Cikarma.. : Sum  Inputs=+-  OutDataType=fixdt(1, 16)  OutScaling=2^-10
  Data Type Conversion : DataTypeConversion  OutDataTypeMode=double  OutDataType=fixdt(1, 16)  OutScaling=2^0
  Data Type Conversion1 : DataTypeConversion  OutDataTypeMode=double  OutDataType=fixdt(1, 16)  OutScaling=2^0
  Data Type Conversion3 : DataTypeConversion  OutDataTypeMode=double  OutDataType=fixdt(1, 16)  OutScaling=2^0
  Dinamik direnc bolucu : Constant  Value=2.0408  OutDataType=fixdt(1, 16)  OutScaling=2^0
  Dinamik port bayasi : Constant  Value=185.00  OutDataType=fixdt(1, 16)  OutScaling=2^0
  Kelvin : Constant  Value=273.00  OutDataType=fixdt(1, 16)  OutScaling=2^0
  Sicaklik Carpani : Constant  Value=0.1  OutDataType=fixdt(1, 16)  OutScaling=2^0
  Statik direnc bolucu : Constant  Value=1.99558  OutDataType=fixdt(1, 16)  OutScaling=2^0
  Statik port bayasi : Constant  Value=200.00  OutDataType=fixdt(1, 16)  OutScaling=2^0
  Sicaklik : Outport  OutDataType=fixdt(1, 16)  OutScaling=2^0
  Statik basinc : Outport  Port=2  OutDataType=fixdt(1, 16)  OutScaling=2^0
  Fark basinc : Outport  Port=3  OutDataType=fixdt(1, 16)  OutScaling=2^0
  wires:
  Carpma/1 -> Cikarma/1
  Kelvin/1 -> Cikarma/2
  Cikarma/1 -> Sicaklik/1
  Data Type Conversion3/1 -> Carpma/1
  RAWtemp/1 -> Data Type Conversion3/1
  Bit agirligi1/1 -> Carpma/2
  Sicaklik Carpani/1 -> Carpma/3
  RAW Diff/1 -> Data Type Conversion/1
  Dinamik direnc bolucu/1 -> Carpma../2
  Bit agirligi./1 -> Carpma../3
  Carpma../1 -> Cikarma../1
  Dinamik port bayasi/1 -> Cikarma../2
  Cikarma../1 -> 1/Hassasiyet1/1
  Data Type Conversion/1 -> Carpma../1
  1/Hassasiyet1/1 -> Fark basinc/1
  RAW Static/1 -> Data Type Conversion1/1
  Statik direnc bolucu/1 -> Carpma./2
  Bit agirligi/1 -> Carpma./3
  Carpma./1 -> Cikarma./1
  Statik port bayasi/1 -> Cikarma./2
  Cikarma./1 -> 1/Hassasiyet/1
  1/Hassasiyet/1 -> Statik basinc/1
  Data Type Conversion1/1 -> Carpma./1

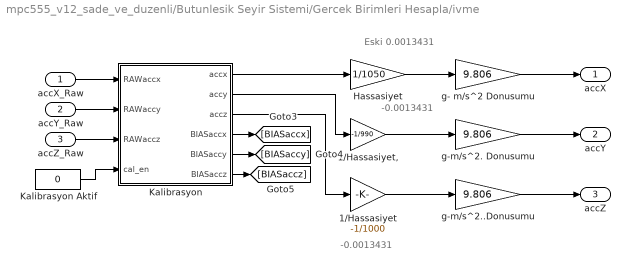
== system mpc555_v12_sade_ve_duzenli/Butunlesik Seyir Sistemi/Gercek Birimleri Hesapla/ivme ==
  note: Eski 0.0013431
  note: -0.0013431
  note: -0.0013431
  accX_Raw : Inport  OutDataType=sfix(16)  OutScaling=2^0
  accY_Raw : Inport  Port=2  OutDataType=sfix(16)  OutScaling=2^0
  accZ_Raw : Inport  Port=3  OutDataType=sfix(16)  OutScaling=2^0
  1/Hassasiyet : Gain  Gain=-1/1000  ParameterDataType=fixdt(1, 16)  ParameterScaling=2^0  OutDataType=fixdt(1, 16)  OutScaling=2^0  SampleTime=dt
  1/Hassasiyet, : Gain  Gain=-1/990  ParameterDataType=fixdt(1, 16)  ParameterScaling=2^0  OutDataType=fixdt(1, 16)  OutScaling=2^0  SampleTime=dt
  Hassasiyet : Gain  Gain=1/1050  ParameterDataType=fixdt(1, 16)  ParameterScaling=2^0  OutDataType=fixdt(1, 16)  OutScaling=2^0  SampleTime=dt
  Kalibrasyon : Stateflow chart  TreatAsAtomicUnit=on
  Kalibrasyon Aktif : Constant  Value=0  OutDataType=fixdt(1, 16)  OutScaling=2^0
  g- m/s^2 Donusumu : Gain  Gain=9.806  ParameterDataType=fixdt(1, 16)  ParameterScaling=2^0  OutDataType=fixdt(1, 16)  OutScaling=2^0  SampleTime=dt
  g-m/s^2. Donusumu : Gain  Gain=9.806  ParameterDataType=fixdt(1, 16)  ParameterScaling=2^0  OutDataType=fixdt(1, 16)  OutScaling=2^0  SampleTime=dt
  g-m/s^2..Donusumu : Gain  Gain=9.806  ParameterDataType=fixdt(1, 16)  ParameterScaling=2^0  OutDataType=fixdt(1, 16)  OutScaling=2^0  SampleTime=dt
  accX : Outport  OutDataType=fixdt(1, 16)  OutScaling=2^0
  accY : Outport  Port=2  OutDataType=fixdt(1, 16)  OutScaling=2^0
  accZ : Outport  Port=3  OutDataType=fixdt(1, 16)  OutScaling=2^0
  wires:
  1/Hassasiyet/1 -> g-m/s^2..Donusumu/1
  1/Hassasiyet,/1 -> g-m/s^2. Donusumu/1
  Hassasiyet/1 -> g- m/s^2 Donusumu/1
  Kalibrasyon/4(BIASaccx) -> [BIASaccx]
  Kalibrasyon/5(BIASaccy) -> [BIASaccy]
  Kalibrasyon/6(BIASaccz) -> [BIASaccz]
  Kalibrasyon Aktif/1 -> Kalibrasyon/4(cal_en)
  accX_Raw/1 -> Kalibrasyon/1(RAWaccx)
  accY_Raw/1 -> Kalibrasyon/2(RAWaccy)
  accZ_Raw/1 -> Kalibrasyon/3(RAWaccz)
  Kalibrasyon/1(accx) -> Hassasiyet/1
  Kalibrasyon/2(accy) -> 1/Hassasiyet,/1
  Kalibrasyon/3(accz) -> 1/Hassasiyet/1
  g- m/s^2 Donusumu/1 -> accX/1
  g-m/s^2. Donusumu/1 -> accY/1
  g-m/s^2..Donusumu/1 -> accZ/1

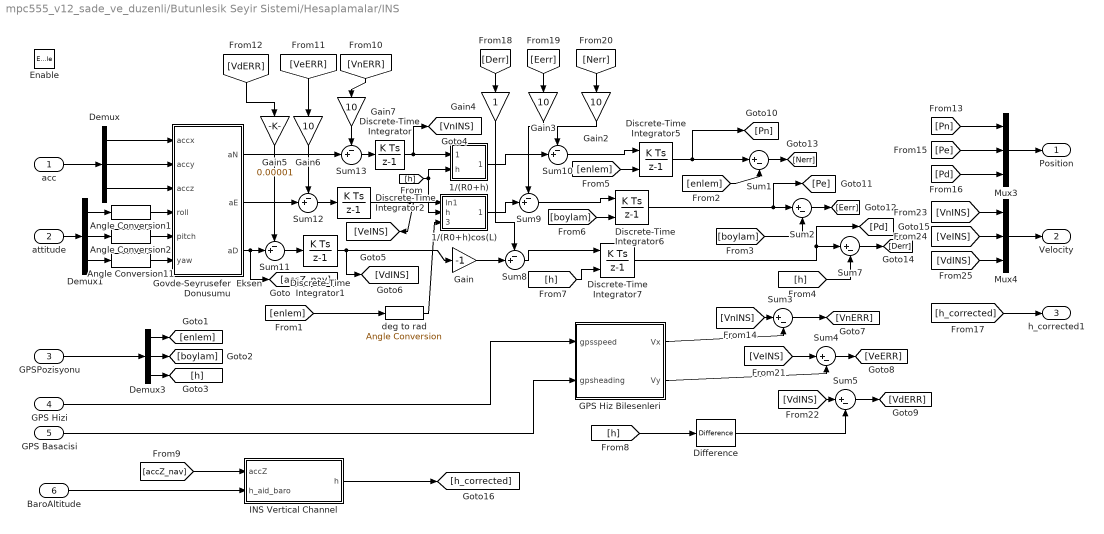
== system mpc555_v12_sade_ve_duzenli/Butunlesik Seyir Sistemi/Hesaplamalar/INS ==
  acc : Inport  OutDataType=sfix(16)  OutScaling=2^0
  attitude : Inport  Port=2  OutDataType=sfix(16)  OutScaling=2^0
  GPSPozisyonu : Inport  Port=3  OutDataType=sfix(16)  OutScaling=2^0
  GPS Hizi : Inport  Port=4  OutDataType=sfix(16)  OutScaling=2^0
  GPS Basacisi : Inport  Port=5  OutDataType=sfix(16)  OutScaling=2^0
  BaroAltitude : Inport  Port=6  OutDataType=sfix(16)  OutScaling=2^0
  Enable : EnablePort
  1/(R0+h) : Subsystem
  1/(R0+h)cos(L) : Subsystem
  Angle Conversion1 : aerolibconvert2/Angle Conversion  SystemSampleTime=-1  IU=deg  OU=rad
  Angle Conversion11 : aerolibconvert2/Angle Conversion  SystemSampleTime=-1  IU=deg  OU=rad
  Angle Conversion2 : aerolibconvert2/Angle Conversion  SystemSampleTime=-1  IU=deg  OU=rad
  Demux : Demux  Outputs=3
  Demux1 : Demux  Outputs=3
  Demux3 : Demux  Outputs=3
  Difference : simulink/Discrete/Difference  SystemSampleTime=-1  ICPrevInput=0.0  OutMin=[]  OutMax=[]  OutDataType=fixdt(1, 16)  OutScaling=2^-10  DoSatur=off
  Discrete-Time Integrator : DiscreteIntegrator  SampleTime=dt  OutDataType=sfix(16)  OutScaling=2^0  ICPrevOutput=DiscIntNeverNeededParam  ICPrevScaledInput=DiscIntNeverNeededParam
  Discrete-Time Integrator1 : DiscreteIntegrator  SampleTime=dt  OutDataType=sfix(16)  OutScaling=2^0  ICPrevOutput=DiscIntNeverNeededParam  ICPrevScaledInput=DiscIntNeverNeededParam
  Discrete-Time Integrator2 : DiscreteIntegrator  SampleTime=dt  OutDataType=sfix(16)  OutScaling=2^0  ICPrevOutput=DiscIntNeverNeededParam  ICPrevScaledInput=DiscIntNeverNeededParam
  Discrete-Time Integrator5 : DiscreteIntegrator  InitialConditionSource=external  SampleTime=dt  OutDataType=sfix(16)  OutScaling=2^0  ICPrevOutput=DiscIntNeverNeededParam  ICPrevScaledInput=DiscIntNeverNeededParam
  Discrete-Time Integrator6 : DiscreteIntegrator  InitialConditionSource=external  SampleTime=dt  OutDataType=sfix(16)  OutScaling=2^0  ICPrevOutput=DiscIntNeverNeededParam  ICPrevScaledInput=DiscIntNeverNeededParam
  Discrete-Time Integrator7 : DiscreteIntegrator  InitialConditionSource=external  SampleTime=dt  OutDataType=sfix(16)  OutScaling=2^0  ICPrevOutput=DiscIntNeverNeededParam  ICPrevScaledInput=DiscIntNeverNeededParam
  GPS Hiz Bilesenleri : Stateflow chart  TreatAsAtomicUnit=on
  Gain : Gain  Gain=-1  ParameterDataType=fixdt(1, 16)  ParameterScaling=2^0  OutDataType=fixdt(1, 16)  OutScaling=2^0
  Gain{2..3,6..7} (4 alike) : Gain  Orientation=down  Gain=10  ParameterDataType=fixdt(1, 16)  ParameterScaling=2^0  OutDataType=fixdt(1, 16)  OutScaling=2^0  SampleTime=dt
  Gain4 : Gain  Orientation=down  ParameterDataType=fixdt(1, 16)  ParameterScaling=2^0  OutDataType=fixdt(1, 16)  OutScaling=2^0  SampleTime=dt
  Gain5 : Gain  Orientation=down  Gain=0.00001  ParameterDataType=fixdt(1, 16)  ParameterScaling=2^0  OutDataType=fixdt(1, 16)  OutScaling=2^0  SampleTime=dt
  Govde-Seyrusefer  Eksen Donusumu : Stateflow chart  TreatAsAtomicUnit=on
  INS Vertical Channel : Subsystem
  Mux3 : Mux  Inputs=3
  Mux4 : Mux  Inputs=3
  Sum{1..5,7} (6 alike) : Sum  Inputs=|+-  OutDataType=fixdt(1, 16)  OutScaling=2^0
  Sum{8..13} (6 alike) : Sum  Inputs=-+|  OutDataType=fixdt(1, 16)  OutScaling=2^0
  deg to rad : aerolibconvert2/Angle Conversion  SystemSampleTime=-1  IU=deg  OU=rad
  Position : Outport  OutDataType=sfix(16)  OutScaling=2^0
  Velocity : Outport  Port=2  OutDataType=sfix(16)  OutScaling=2^0
  h_corrected1 : Outport  Port=3  OutDataType=sfix(16)  OutScaling=2^0
  wires:
  Difference/1 -> Sum5/2
  GPS Hiz Bilesenleri/2(Vy) -> Sum4/2
  GPS Hiz Bilesenleri/1(Vx) -> Sum3/2
  [h] -> Difference/1
  GPS Hizi/1 -> GPS Hiz Bilesenleri/1(gpsspeed)
  GPS Basacisi/1 -> GPS Hiz Bilesenleri/2(gpsheading)
  [h] -> Discrete-Time Integrator7/2
  [boylam] -> Discrete-Time Integrator6/2
  [enlem] -> Discrete-Time Integrator5/2
  [boylam] -> Sum2/2
  [h] -> Sum7/2
  [enlem] -> Sum1/2
  Demux3/3 -> [h]
  Demux3/2 -> [boylam]
  [enlem] -> deg to rad/1
  Demux3/1 -> [enlem]
  GPSPozisyonu/1 -> Demux3/1
  [Derr] -> Gain4/1
  [Nerr] -> Gain2/1
  [Eerr] -> Gain3/1
  Discrete-Time Integrator7/1 -> Sum7/1, [Pd]
  Discrete-Time Integrator6/1 -> Sum2/1, [Pe]
  Discrete-Time Integrator5/1 -> Sum1/1, [Pn]
  Demux1/3 -> Angle Conversion11/1
  Gain/1 -> Sum8/2
  1/(R0+h)cos(L)/1(Out1) -> Sum9/2
  Discrete-Time Integrator2/1 -> 1/(R0+h)cos(L)/1(In1), [VeINS]
  deg to rad/1 -> 1/(R0+h)cos(L)/3(enlem)
  [h] -> 1/(R0+h)cos(L)/2(h), 1/(R0+h)/2(h)
  1/(R0+h)/1(Out1) -> Sum10/2
  Demux1/2 -> Angle Conversion2/1
  Demux1/1 -> Angle Conversion1/1
  attitude/1 -> Demux1/1
  acc/1 -> Demux/1
  Demux/3 -> Govde-Seyrusefer  Eksen Donusumu/3(accz)
  Demux/2 -> Govde-Seyrusefer  Eksen Donusumu/2(accy)
  Demux/1 -> Govde-Seyrusefer  Eksen Donusumu/1(accx)
  Sum7/1 -> [Derr]
  Sum2/1 -> [Eerr]
  Sum1/1 -> [Nerr]
  [VnERR] -> Gain7/1
  [VdERR] -> Gain5/1
  Sum9/1 -> Discrete-Time Integrator6/1
  Gain5/1 -> Sum11/1
  Gain6/1 -> Sum12/1
  Gain7/1 -> Sum13/1
  Sum11/1 -> Discrete-Time Integrator1/1
  Sum12/1 -> Discrete-Time Integrator2/1
  Govde-Seyrusefer  Eksen Donusumu/2(aE) -> Sum12/2
  Sum13/1 -> Discrete-Time Integrator/1
  Govde-Seyrusefer  Eksen Donusumu/1(aN) -> Sum13/2
  Gain3/1 -> Sum9/1
  Gain2/1 -> Sum10/1
  Sum8/1 -> Discrete-Time Integrator7/1
  Sum10/1 -> Discrete-Time Integrator5/1
  Angle Conversion11/1 -> Govde-Seyrusefer  Eksen Donusumu/6(yaw)
  Angle Conversion2/1 -> Govde-Seyrusefer  Eksen Donusumu/5(pitch)
  Angle Conversion1/1 -> Govde-Seyrusefer  Eksen Donusumu/4(roll)
  Discrete-Time Integrator1/1 -> Gain/1, [VdINS]
  Govde-Seyrusefer  Eksen Donusumu/3(aD) -> Sum11/2, [accZ_nav]
  INS Vertical Channel/1(h) -> [h_corrected]
  BaroAltitude/1 -> INS Vertical Channel/2(h_aid_baro)
  [accZ_nav] -> INS Vertical Channel/1(accZ)
  [VnINS] -> Sum3/1
  [VeINS] -> Sum4/1
  [VdINS] -> Sum5/1
  Sum3/1 -> [VnERR]
  Sum4/1 -> [VeERR]
  Sum5/1 -> [VdERR]
  [VeERR] -> Gain6/1
  Mux3/1 -> Position/1
  Mux4/1 -> Velocity/1
  [h_corrected] -> h_corrected1/1
  [Pn] -> Mux3/1
  [Pe] -> Mux3/2
  [Pd] -> Mux3/3
  [VnINS] -> Mux4/1
  [VeINS] -> Mux4/2
  [VdINS] -> Mux4/3
  Gain4/1 -> Sum8/1
  Discrete-Time Integrator/1 -> 1/(R0+h)/1(In1), [VnINS]

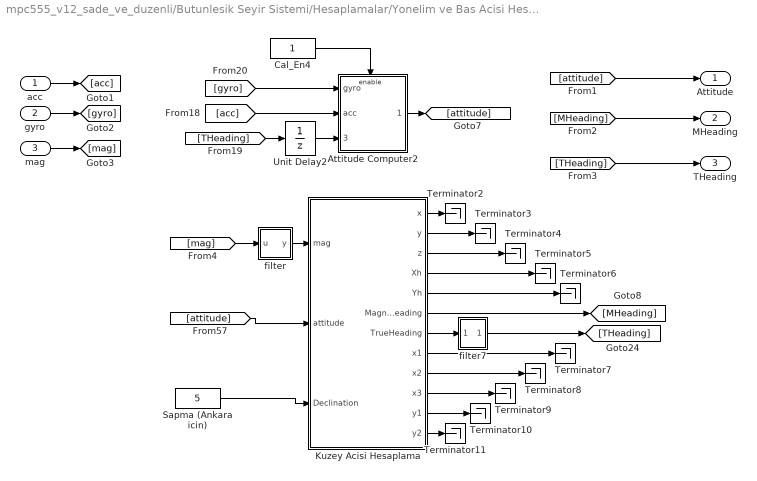
== system mpc555_v12_sade_ve_duzenli/Butunlesik Seyir Sistemi/Hesaplamalar/Yonelim ve Bas Acisi Hesaplama ==
  acc : Inport  OutDataType=fixdt(1, 16)  OutScaling=2^0
  gyro : Inport  Port=2  OutDataType=fixdt(1, 16)  OutScaling=2^0
  mag : Inport  Port=3  OutDataType=fixdt(1, 16)  OutScaling=2^0
  Attitude Computer2 : Subsystem
  Cal_En4 : Constant  OutDataType=fixdt(1, 16)  OutScaling=2^0
  Kuzey Acisi Hesaplama : Stateflow chart  TreatAsAtomicUnit=on
  "Sapma (Ankara icin) " : Constant  Value=5  OutDataType=fixdt(1, 16)  OutScaling=2^0
  Terminator{2..11} (10 alike) : Terminator
  Unit Delay2 : UnitDelay  SampleTime=-1
  filter : Stateflow chart  TreatAsAtomicUnit=on
  filter7 : Stateflow chart  TreatAsAtomicUnit=on
  Attitude : Outport  OutDataType=fixdt(1, 16)  OutScaling=2^0
  MHeading : Outport  Port=2  OutDataType=fixdt(1, 16)  OutScaling=2^0
  THeading : Outport  Port=3  OutDataType=fixdt(1, 16)  OutScaling=2^0
  wires:
  Unit Delay2/1 -> Attitude Computer2/3(TrueHeading)
  [THeading] -> Unit Delay2/1
  [acc] -> Attitude Computer2/2(acc)
  [gyro] -> Attitude Computer2/1(gyro)
  Attitude Computer2/1(attitude) -> [attitude]
  Cal_En4/1 -> Attitude Computer2/Enable
  [attitude] -> Kuzey Acisi Hesaplama/2(attitude)
  "Sapma (Ankara icin) "/1 -> Kuzey Acisi Hesaplama/3(Declination)
  Kuzey Acisi Hesaplama/7(TrueHeading) -> filter7/1(u)
  Kuzey Acisi Hesaplama/6(MagneticHeading) -> [MHeading]
  [mag] -> filter/1(u)
  filter/1(y) -> Kuzey Acisi Hesaplama/1(mag)
  filter7/1(y) -> [THeading]
  [attitude] -> Attitude/1
  [MHeading] -> MHeading/1
  [THeading] -> THeading/1
  acc/1 -> [acc]
  gyro/1 -> [gyro]
  mag/1 -> [mag]
  Kuzey Acisi Hesaplama/1(x) -> Terminator2/1
  Kuzey Acisi Hesaplama/2(y) -> Terminator3/1
  Kuzey Acisi Hesaplama/3(z) -> Terminator4/1
  Kuzey Acisi Hesaplama/4(Xh) -> Terminator5/1
  Kuzey Acisi Hesaplama/5(Yh) -> Terminator6/1
  Kuzey Acisi Hesaplama/8(x1) -> Terminator7/1
  Kuzey Acisi Hesaplama/9(x2) -> Terminator8/1
  Kuzey Acisi Hesaplama/10(x3) -> Terminator9/1
  Kuzey Acisi Hesaplama/11(y1) -> Terminator10/1
  Kuzey Acisi Hesaplama/12(y2) -> Terminator11/1

== system mpc555_v12_sade_ve_duzenli/Butunlesik Seyir Sistemi/Hesaplamalar/INS/1/(R0+h) ==
  In1 : Inport  OutDataType=fixdt(1, 16)  OutScaling=2^0
  h : Inport  Port=2  OutDataType=fixdt(1, 16)  OutScaling=2^0
  Divide : Product  Inputs=*/  OutDataType=fixdt(1, 16)  OutScaling=2^-10  SampleTime=dt
  R0(m) : Constant  Value=6378000  OutDataTypeMode=double  OutDataType=fixdt(1, 16)  OutScaling=2^0  SampleTime=dt
  Sum : Sum  Inputs=|++  OutDataType=fixdt(1, 16)  OutScaling=2^0
  Out1 : Outport  OutDataType=fixdt(1, 16)  OutScaling=2^0
  wires:
  In1/1 -> Divide/1
  Divide/1 -> Out1/1
  Sum/1 -> Divide/2
  R0(m)/1 -> Sum/2
  h/1 -> Sum/1

== system mpc555_v12_sade_ve_duzenli/Butunlesik Seyir Sistemi/Hesaplamalar/INS/1/(R0+h)cos(L) ==
  In1 : Inport  OutDataType=fixdt(1, 16)  OutScaling=2^0
  h : Inport  Port=2  OutDataType=fixdt(1, 16)  OutScaling=2^0
  enlem : Inport  Port=3  OutDataType=fixdt(1, 16)  OutScaling=2^0
  Divide : Product  Inputs=*/  OutDataType=fixdt(1, 16)  OutScaling=2^-10
  Product : Product  OutDataType=fixdt(1, 16)  OutScaling=2^0  RndMeth=Zero
  R0(m) : Constant  Value=6378000  OutDataTypeMode=double  OutDataType=fixdt(1, 16)  OutScaling=2^0
  Sum : Sum  Inputs=|++  OutDataType=fixdt(1, 16)  OutScaling=2^0
  Trigonometric Function : Trigonometry  Operator=cos
  Out1 : Outport  OutDataType=fixdt(1, 16)  OutScaling=2^0
  wires:
  Trigonometric Function/1 -> Product/2
  Product/1 -> Divide/2
  enlem/1 -> Trigonometric Function/1
  Sum/1 -> Product/1
  h/1 -> Sum/1
  R0(m)/1 -> Sum/2
  Divide/1 -> Out1/1
  In1/1 -> Divide/1

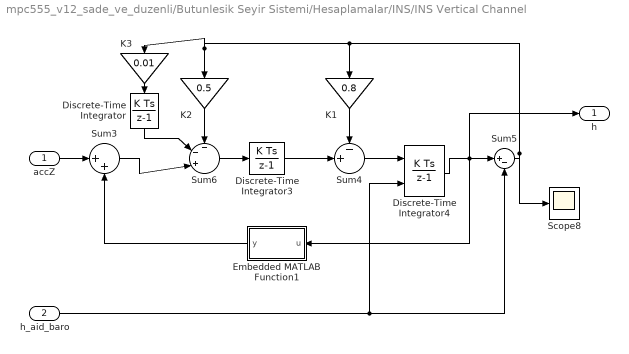
== system mpc555_v12_sade_ve_duzenli/Butunlesik Seyir Sistemi/Hesaplamalar/INS/INS Vertical Channel ==
  accZ : Inport  OutDataType=fixdt(1, 16)  OutScaling=2^0
  h_aid_baro : Inport  Port=2  OutDataType=sfix(16)  OutScaling=2^0
  Discrete-Time Integrator : DiscreteIntegrator  Orientation=down  SampleTime=dt  OutDataType=sfix(16)  OutScaling=2^0  ICPrevOutput=DiscIntNeverNeededParam  ICPrevScaledInput=DiscIntNeverNeededParam
  Discrete-Time Integrator3 : DiscreteIntegrator  SampleTime=dt  OutDataType=sfix(16)  OutScaling=2^0  ICPrevOutput=DiscIntNeverNeededParam  ICPrevScaledInput=DiscIntNeverNeededParam
  Discrete-Time Integrator4 : DiscreteIntegrator  InitialConditionSource=external  SampleTime=dt  OutDataType=sfix(16)  OutScaling=2^0  ICPrevOutput=DiscIntNeverNeededParam  ICPrevScaledInput=DiscIntNeverNeededParam
  Embedded MATLAB Function1 : Stateflow chart  Orientation=left  TreatAsAtomicUnit=on
  K1 : Gain  Orientation=down  Gain=0.8  ParameterDataType=fixdt(1, 16)  ParameterScaling=2^0  OutDataType=fixdt(1, 16)  OutScaling=2^0
  K2 : Gain  Orientation=down  Gain=0.5  ParameterDataType=fixdt(1, 16)  ParameterScaling=2^0  OutDataType=fixdt(1, 16)  OutScaling=2^0
  K3 : Gain  Orientation=down  Gain=0.01  ParameterDataType=fixdt(1, 16)  ParameterScaling=2^0  OutDataType=fixdt(1, 16)  OutScaling=2^0
  Scope8 : Scope
      settings: TimeRange=10  YMin=-60  YMax=20  SaveName=ScopeData26
  Sum3 : Sum  Inputs=|++  OutDataType=fixdt(1, 16)  OutScaling=2^0
  Sum4 : Sum  Inputs=-+|  OutDataType=fixdt(1, 16)  OutScaling=2^0
  Sum5 : Sum  Inputs=|+-  OutDataType=fixdt(1, 16)  OutScaling=2^0
  Sum6 : Sum  Inputs=--+|  OutDataType=fixdt(1, 16)  OutScaling=2^0
  h : Outport  OutDataType=sfix(16)  OutScaling=2^0
  wires:
  K3/1 -> Discrete-Time Integrator/1
  Discrete-Time Integrator/1 -> Sum6/2
  Sum3/1 -> Sum6/3
  accZ/1 -> Sum3/1
  h_aid_baro/1 -> Sum5/2, Discrete-Time Integrator4/2
  K1/1 -> Sum4/1
  K2/1 -> Sum6/1
  Embedded MATLAB Function1/1(y) -> Sum3/2
  Sum6/1 -> Discrete-Time Integrator3/1
  Sum5/1 -> K3/1, K2/1, K1/1, Scope8/1
  Discrete-Time Integrator3/1 -> Sum4/2
  Discrete-Time Integrator4/1 -> h/1, Embedded MATLAB Function1/1(u), Sum5/1
  Sum4/1 -> Discrete-Time Integrator4/1

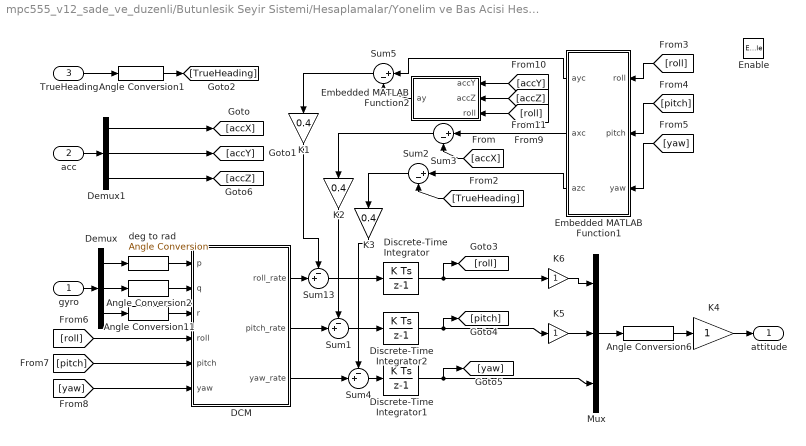
== system mpc555_v12_sade_ve_duzenli/Butunlesik Seyir Sistemi/Hesaplamalar/Yonelim ve Bas Acisi Hesaplama/Attitude Computer2 ==
  gyro : Inport  OutDataType=sfix(16)  OutScaling=2^0
  acc : Inport  Port=2  OutDataType=sfix(16)  OutScaling=2^0
  TrueHeading : Inport  Port=3  OutDataType=sfix(16)  OutScaling=2^0
  Enable : EnablePort  StatesWhenEnabling=reset
  Angle Conversion1 : aerolibconvert2/Angle Conversion  SystemSampleTime=-1  IU=deg  OU=rad
  Angle Conversion11 : aerolibconvert2/Angle Conversion  SystemSampleTime=-1  IU=deg  OU=rad
  Angle Conversion2 : aerolibconvert2/Angle Conversion  SystemSampleTime=-1  IU=deg  OU=rad
  Angle Conversion6 : aerolibconvert2/Angle Conversion  SystemSampleTime=-1  IU=rad  OU=deg
  DCM : Stateflow chart  TreatAsAtomicUnit=on
  Demux : Demux  Outputs=3
  Demux1 : Demux  Outputs=3
  Discrete-Time Integrator : DiscreteIntegrator  gainval=1  SampleTime=dt  OutDataType=sfix(16)  OutScaling=2^0  LimitOutput=on  UpperSaturationLimit=3.14  LowerSaturationLimit=-3.14  ICPrevOutput=DiscIntNeverNeededParam  ICPrevScaledInput=DiscIntNeverNeededParam
  Discrete-Time Integrator1 : DiscreteIntegrator  InitialConditionMode=State only (most efficient)  SampleTime=dt  OutDataType=sfix(16)  OutScaling=2^0  ICPrevOutput=DiscIntNeverNeededParam  ICPrevScaledInput=DiscIntNeverNeededParam
  Discrete-Time Integrator2 : DiscreteIntegrator  gainval=1  SampleTime=dt  OutDataType=sfix(16)  OutScaling=2^0  LimitOutput=on  UpperSaturationLimit=1.53  LowerSaturationLimit=-1.53  ICPrevOutput=DiscIntNeverNeededParam  ICPrevScaledInput=DiscIntNeverNeededParam
  Embedded MATLAB Function1 : Stateflow chart  Orientation=left  TreatAsAtomicUnit=on
  Embedded MATLAB Function2 : Stateflow chart  Orientation=left  TreatAsAtomicUnit=on
  K1 : Gain  Orientation=down  Gain=0.4  ParameterDataType=fixdt(1, 16)  ParameterScaling=2^0  OutDataType=fixdt(1, 16)  OutScaling=2^0  SampleTime=dt
  K2 : Gain  Orientation=down  Gain=0.4  ParameterDataType=fixdt(1, 16)  ParameterScaling=2^0  OutDataType=fixdt(1, 16)  OutScaling=2^0  SampleTime=dt
  K3 : Gain  Orientation=down  Gain=0.4  ParameterDataType=fixdt(1, 16)  ParameterScaling=2^0  OutDataType=fixdt(1, 16)  OutScaling=2^0  SampleTime=dt
  K4 : Gain  ParameterDataType=fixdt(1, 16)  ParameterScaling=2^0  OutDataType=fixdt(1, 16)  OutScaling=2^0  SampleTime=dt
  K5 : Gain  ParameterDataType=fixdt(1, 16)  ParameterScaling=2^0  OutDataType=fixdt(1, 16)  OutScaling=2^0  SampleTime=dt
  K6 : Gain  ParameterDataType=fixdt(1, 16)  ParameterScaling=2^0  OutDataType=fixdt(1, 16)  OutScaling=2^0  SampleTime=dt
  Mux : Mux  Inputs=3
  Sum1 : Sum  Inputs=-+|  OutDataType=fixdt(1, 16)  OutScaling=2^0
  Sum13 : Sum  Inputs=-+|  OutDataType=fixdt(1, 16)  OutScaling=2^0
  Sum2 : Sum  Orientation=left  Inputs=|+-  OutDataType=fixdt(1, 16)  OutScaling=2^0
  Sum3 : Sum  Orientation=left  Inputs=|+-  OutDataType=fixdt(1, 16)  OutScaling=2^0
  Sum4 : Sum  Inputs=-+|  OutDataType=fixdt(1, 16)  OutScaling=2^0
  Sum5 : Sum  Orientation=left  Inputs=|+-  OutDataType=fixdt(1, 16)  OutScaling=2^0
  deg to rad : aerolibconvert2/Angle Conversion  SystemSampleTime=-1  IU=deg  OU=rad
  attitude : Outport  OutDataType=sfix(16)  OutScaling=2^0
  wires:
  TrueHeading/1 -> Angle Conversion1/1
  Angle Conversion11/1 -> DCM/3(r)
  Angle Conversion2/1 -> DCM/2(q)
  deg to rad/1 -> DCM/1(p)
  Discrete-Time Integrator2/1 -> [pitch], K5/1
  Discrete-Time Integrator1/1 -> Mux/3, [yaw]
  Demux/1 -> deg to rad/1
  Demux/2 -> Angle Conversion2/1
  Demux/3 -> Angle Conversion11/1
  gyro/1 -> Demux/1
  acc/1 -> Demux1/1
  Mux/1 -> Angle Conversion6/1
  K1/1 -> Sum13/1
  K2/1 -> Sum1/1
  K3/1 -> Sum4/1
  DCM/1(roll_rate) -> Sum13/2
  DCM/2(pitch_rate) -> Sum1/2
  DCM/3(yaw_rate) -> Sum4/2
  Sum13/1 -> Discrete-Time Integrator/1
  Sum1/1 -> Discrete-Time Integrator2/1
  Sum4/1 -> Discrete-Time Integrator1/1
  Sum5/1 -> K1/1
  Sum3/1 -> K2/1
  Sum2/1 -> K3/1
  Demux1/1 -> [accX]
  Demux1/2 -> [accY]
  [accX] -> Sum3/2
  Angle Conversion1/1 -> [TrueHeading]
  [TrueHeading] -> Sum2/2
  Embedded MATLAB Function1/2(axc) -> Sum3/1
  Embedded MATLAB Function1/1(ayc) -> Sum5/1
  Embedded MATLAB Function1/3(azc) -> Sum2/1
  Discrete-Time Integrator/1 -> K6/1, [roll]
  Angle Conversion6/1 -> K4/1
  [pitch] -> Embedded MATLAB Function1/2(pitch)
  [yaw] -> Embedded MATLAB Function1/3(yaw)
  [roll] -> DCM/4(roll)
  [pitch] -> DCM/5(pitch)
  [yaw] -> DCM/6(yaw)
  K4/1 -> attitude/1
  K5/1 -> Mux/2
  K6/1 -> Mux/1
  [roll] -> Embedded MATLAB Function2/3(roll)
  [accY] -> Embedded MATLAB Function2/1(accY)
  [accZ] -> Embedded MATLAB Function2/2(accZ)
  Embedded MATLAB Function2/1(ay) -> Sum5/2
  Demux1/3 -> [accZ]
  [roll] -> Embedded MATLAB Function1/1(roll)
